simulink model "question7"  (R2018a)
settings: Solver=FixedStepAuto  StartTime=0.0  StopTime=10.0  FixedStep=0.001  RelTol=1e-3
settings Model: Creator=arjun  LastModifiedBy=arjun

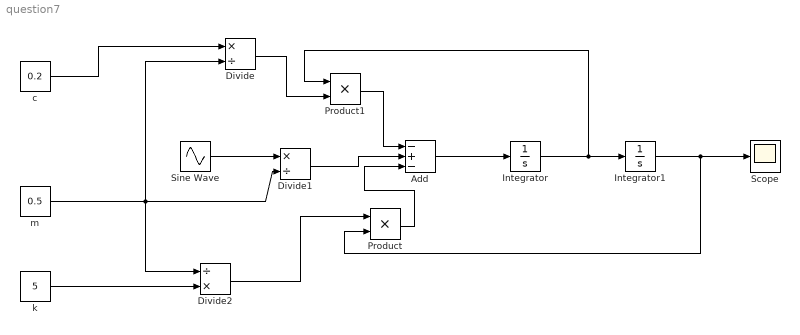
== system question7 ==
  Add : Sum  Inputs=-+-
  Divide : Product  Inputs=*/
  Divide1 : Product  Inputs=*/
  Divide2 : Product  Inputs=/*
  Integrator : Integrator
  Integrator1 : Integrator  InitialCondition=0.000025
  Product : Product
  Product1 : Product
  Scope : Scope
  Sine Wave : Sin  Amplitude=2  Frequency=50  SampleTime=0
  c : Constant  Value=0.2
  k : Constant  Value=5
  m : Constant  Value=0.5
  wires:
  k/1 -> Divide2/2
  Sine Wave/1 -> Divide1/1
  m/1 -> Divide/2, Divide1/2, Divide2/1
  c/1 -> Divide/1
  Divide2/1 -> Product/1
  Divide1/1 -> Add/2
  Product/1 -> Add/3
  Product1/1 -> Add/1
  Divide/1 -> Product1/2
  Add/1 -> Integrator/1
  Integrator/1 -> Product1/1, Integrator1/1
  Integrator1/1 -> Product/2, Scope/1
